simulink model "FKtestZERO"  (Simulink 6.6)
settings: Solver=ode4  StartTime=0.0  StopTime=400  FixedStep=0.05  RelTol=1e-3
libraries: marine_gnc x2, simulink x1, hydro x1
settings Model: Creator=Thor  LastModifiedBy=Thor

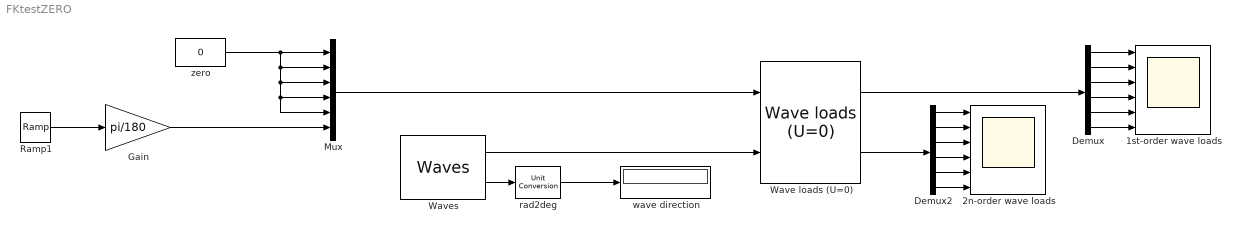
== system FKtestZERO ==
  "1st-order wave loads " : Scope  NumInputPorts=6
      settings: TimeRange=250  YMin=-4000000~-10000000~-40000000~-10000000~-400000000~-100000000  YMax=4000000~10000000~40000000~10000000~400000000~100000000
  2n-order wave loads : Scope  NumInputPorts=6
      settings: TimeRange=400  YMin=-60000~-400000~-1~-1~-1~200000  YMax=20000~400000~1~1~1~1000000
  Demux : Demux  Outputs=6
  Demux2 : Demux  Outputs=6
  Gain : Gain  Gain=pi/180
  Mux : Mux  Inputs=6
  Ramp1 : simulink/Sources/Ramp  SystemSampleTime=-1  slope=1  start=0  X0=0
  Wave loads (U=0) : hydro/Hydro Library/Wave loads (U=0)  SystemSampleTime=-1
  Waves : marine_gnc/Environment/Waves/Waves  SystemSampleTime=-1  spectrum_type=ITTC  disp_flag=off  plot_spectrum=off  plot_realization=off  hs=5  omega_peak=-1  psi_mean=0/(180/pi)  gamma=-1  spread=2  depth=inf  nfreq=20  ndir=10  energylim=0.005  freq_cutoff=3  dir_cutoff=0  rand_seed=0  rand_freq=on  rand_dir=on  Zeta_a=0  Omega=0  Phase=0  Wavenum=0  Psi=0
  rad2deg : marine_gnc/Utilities/Math Operations/Unit Conversion  SystemSampleTime=-1  in=rad2deg
  wave direction : Display
  zero : Constant  Value=0
  wires:
  Ramp1/1 -> Gain/1
  Waves/2 -> rad2deg/1
  rad2deg/1 -> wave direction/1
  zero/1 -> Mux/1, Mux/2, Mux/3, Mux/4, Mux/5
  Gain/1 -> Mux/6
  Mux/1 -> Wave loads (U=0)/1
  Waves/1 -> Wave loads (U=0)/2
  Demux/1 -> "1st-order wave loads "/1
  Demux/2 -> "1st-order wave loads "/2
  Demux/3 -> "1st-order wave loads "/3
  Demux/4 -> "1st-order wave loads "/4
  Demux/5 -> "1st-order wave loads "/5
  Demux/6 -> "1st-order wave loads "/6
  Demux2/1 -> 2n-order wave loads/1
  Demux2/2 -> 2n-order wave loads/2
  Demux2/3 -> 2n-order wave loads/3
  Demux2/4 -> 2n-order wave loads/4
  Demux2/5 -> 2n-order wave loads/5
  Demux2/6 -> 2n-order wave loads/6
  Wave loads (U=0)/1 -> Demux/1
  Wave loads (U=0)/2 -> Demux2/1
